simulink model "systemTest"  (R2014a)
settings: Solver=ode45  StartTime=0.0  StopTime=100  RelTol=1e-3
values from neighbouring files (symbols this model uses):
  friX1 = 4    [parameters1.m]
  friX2 = 0.76462    [parameters1.m]
  friY = 8    [parameters1.m]
  friZ = 4    [parameters1.m]
  I = 1/12*m*((2*ry1)^2 + (2*rx1)^2)    (= 7.53502955357)    [parameters1.m]
  inputBound = [minInput maxInput]    [parameters1.m]
  K = [1000 1000 1000 10 10 1 1]    [parameters1.m]
  k1m = 50    [parameters1.m]
  k1x = 100    [parameters1.m]
  k1y = 100    [parameters1.m]
  k2m = 25    [parameters1.m]
  k2x = 60    [parameters1.m]
  k2y = 60    [parameters1.m]
  m = 46.27    [parameters1.m]
  rx1 = rx01    [Minimizer.m]    (also in parameters1.m = -0.635)
  rx2 = rx02    [Minimizer.m]    (also in parameters1.m = -0.635)
  ry1 = ry01    [Minimizer.m]    (also in parameters1.m = 0.2921)
  ry2 = ry02    [Minimizer.m]    (also in parameters1.m = -0.2921)
settings Model: Creator=propagator  LastModifiedBy=propagator

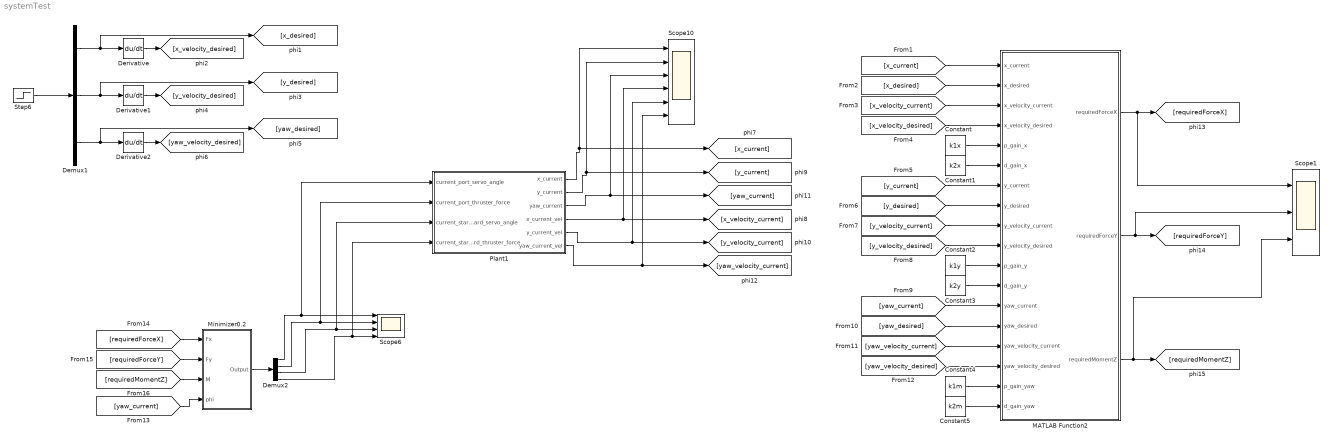
== system systemTest ==
  Constant : Constant  Value=k1x
  Constant1 : Constant  Value=k2x
  Constant2 : Constant  Value=k1y
  Constant3 : Constant  Value=k2y
  Constant4 : Constant  Value=k1m
  Constant5 : Constant  Value=k2m
  Demux1 : Demux  Outputs=3
  Demux2 : Demux
  Derivative : Derivative
  Derivative1 : Derivative
  Derivative2 : Derivative
  MATLAB Function2 : MATLAB Function  TreatAsAtomicUnit=on
  Minimizer0.2 : Subsystem  mask{rx1=rx1, rx2=rx2, ry1=ry1, ry2=ry2, C=K, inputBound=inputBound, m=m, I=I}
      mask prompts: C "Performance Gain"; inputBound "Input Bounds"; m "Boat Mass"; I "Boat Inertia"
      mask TypeOptions m: Constant6/Value
      mask TypeOptions I: Constant7/Value
  Plant1 : Subsystem  mask{rx1=rx1, ry1=ry1, ry2=ry2, M=m, I=I, friX1=friX1, friX2=friX2, friY=friY, friZ=friZ}
      mask TypeOptions rx1: Constant/Value
      mask TypeOptions friX1: Constant1/Value
      mask TypeOptions friX2: Constant8/Value
      mask TypeOptions friY: Constant7/Value
      mask TypeOptions friZ: Constant9/Value
  Scope1 : Scope  NumInputPorts=3
      settings: YMin=-3~905~-185  YMax=0~940~-155
  Scope10 : Scope  NumInputPorts=6
      settings: YMin=1.83~5.87~12~0.03265~0.0811~-0.1116  YMax=1.87~5.97~12.13~0.03305~0.08155~-0.1103  SaveName=ScopeData9
  Scope6 : Scope  NumInputPorts=4
      settings: YMin=-1~-23~45.5556~25  YMax=1~-23~45.5556~32.5  SaveName=ScopeData5
  Step6 : Step  Before=[0;0;0]  After=[0;10;0]  SampleTime=0
  wires:
  Demux2/1 -> Plant1/1(current_port_servo_angle), Scope6/1
  Demux2/2 -> Plant1/2(current_port_thruster_force), Scope6/2
  Demux2/3 -> Plant1/3(current_starboard_servo_angle), Scope6/3
  Demux2/4 -> Plant1/4(current_starboard_thruster_force), Scope6/4
  Minimizer0.2/1(Output) -> Demux2/1
  Constant1/1 -> MATLAB Function2/6(d_gain_x)
  Constant/1 -> MATLAB Function2/5(p_gain_x)
  Constant4/1 -> MATLAB Function2/17(p_gain_yaw)
  Constant5/1 -> MATLAB Function2/18(d_gain_yaw)
  Constant3/1 -> MATLAB Function2/12(d_gain_y)
  Constant2/1 -> MATLAB Function2/11(p_gain_y)
  [x_current] -> MATLAB Function2/1(x_current)
  [x_desired] -> MATLAB Function2/2(x_desired)
  [x_velocity_current] -> MATLAB Function2/3(x_velocity_current)
  [x_velocity_desired] -> MATLAB Function2/4(x_velocity_desired)
  [yaw_velocity_desired] -> MATLAB Function2/16(yaw_velocity_desired)
  [yaw_velocity_current] -> MATLAB Function2/15(yaw_velocity_current)
  [yaw_desired] -> MATLAB Function2/14(yaw_desired)
  [yaw_current] -> MATLAB Function2/13(yaw_current)
  [y_velocity_desired] -> MATLAB Function2/10(y_velocity_desired)
  [y_velocity_current] -> MATLAB Function2/9(y_velocity_current)
  [y_desired] -> MATLAB Function2/8(y_desired)
  [y_current] -> MATLAB Function2/7(y_current)
  Demux1/3 -> [yaw_desired], Derivative2/1
  Demux1/2 -> [y_desired], Derivative1/1
  Derivative2/1 -> [yaw_velocity_desired]
  Derivative1/1 -> [y_velocity_desired]
  Demux1/1 -> [x_desired], Derivative/1
  Step6/1 -> Demux1/1
  Derivative/1 -> [x_velocity_desired]
  Plant1/1(x_current) -> Scope10/1, [x_current]
  Plant1/2(y_current) -> Scope10/2, [y_current]
  Plant1/6(yaw_current_vel) -> Scope10/6, [yaw_velocity_current]
  Plant1/3(yaw_current) -> Scope10/3, [yaw_current]
  Plant1/4(x_current_vel) -> Scope10/4, [x_velocity_current]
  Plant1/5(y_current_vel) -> Scope10/5, [y_velocity_current]
  MATLAB Function2/2(requiredForceY) -> Scope1/2, [requiredForceY]
  MATLAB Function2/3(requiredMomentZ) -> Scope1/3, [requiredMomentZ]
  MATLAB Function2/1(requiredForceX) -> Scope1/1, [requiredForceX]
  [yaw_current] -> Minimizer0.2/4(phi)
  [requiredMomentZ] -> Minimizer0.2/3(M)
  [requiredForceY] -> Minimizer0.2/2(Fy)
  [requiredForceX] -> Minimizer0.2/1(Fx)

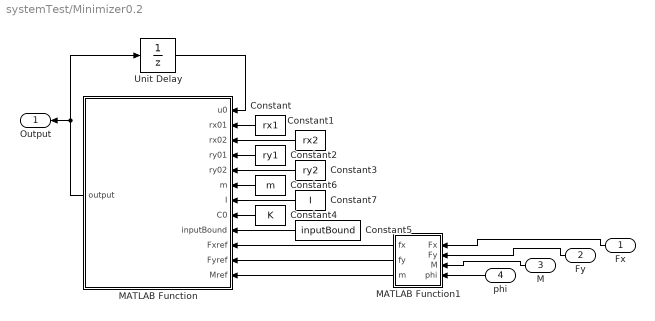
== system systemTest/Minimizer0.2 ==
  Fx : Inport
  Fy : Inport  Port=2
  M : Inport  Port=3
  phi : Inport  Port=4
  Constant : Constant  Value=rx1
  Constant1 : Constant  Value=rx2
  Constant2 : Constant  Value=ry1
  Constant3 : Constant  Value=ry2
  Constant4 : Constant  Value=K
  Constant5 : Constant  Value=inputBound
  Constant6 : Constant  Value=m
  Constant7 : Constant  Value=I
  MATLAB Function : MATLAB Function  TreatAsAtomicUnit=on
  MATLAB Function1 : MATLAB Function  TreatAsAtomicUnit=on
  Unit Delay : UnitDelay  InitialCondition=[0;0;0;0]  SampleTime=-1
  Output : Outport
  wires:
  Constant/1 -> MATLAB Function/2(rx01)
  Constant1/1 -> MATLAB Function/3(rx02)
  Constant2/1 -> MATLAB Function/4(ry01)
  Constant4/1 -> MATLAB Function/8(C0)
  Unit Delay/1 -> MATLAB Function/1(u0)
  MATLAB Function/1(output) -> Unit Delay/1, Output/1
  Constant5/1 -> MATLAB Function/9(inputBound)
  Constant3/1 -> MATLAB Function/5(ry02)
  MATLAB Function1/3(m) -> MATLAB Function/12(Mref)
  MATLAB Function1/2(fy) -> MATLAB Function/11(Fyref)
  MATLAB Function1/1(fx) -> MATLAB Function/10(Fxref)
  Fy/1 -> MATLAB Function1/2(Fy)
  Fx/1 -> MATLAB Function1/1(Fx)
  M/1 -> MATLAB Function1/3(M)
  phi/1 -> MATLAB Function1/4(phi)
  Constant6/1 -> MATLAB Function/6(m)
  Constant7/1 -> MATLAB Function/7(I)

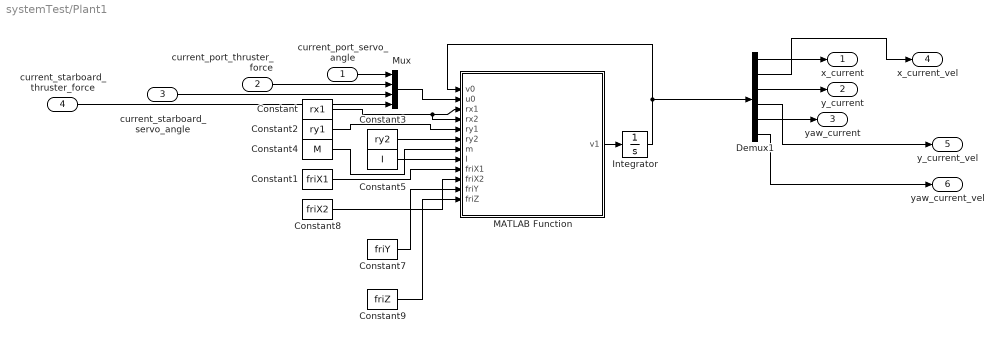
== system systemTest/Plant1 ==
  current_port_servo_angle : Inport
  current_port_thruster_force : Inport  Port=2
  current_starboard_servo_angle : Inport  Port=3
  current_starboard_thruster_force : Inport  Port=4
  Constant : Constant  Value=rx1
  Constant1 : Constant  Value=friX1
  Constant2 : Constant  Value=ry1
  Constant3 : Constant  Value=ry2
  Constant4 : Constant  Value=M
  Constant5 : Constant  Value=I
  Constant7 : Constant  Value=friY
  Constant8 : Constant  Value=friX2
  Constant9 : Constant  Value=friZ
  Demux1 : Demux  Outputs=6
  Integrator : Integrator  InitialCondition=[0 0 0 0 0 0]
  MATLAB Function : MATLAB Function  TreatAsAtomicUnit=on
  Mux : Mux
  x_current : Outport
  y_current : Outport  Port=2
  yaw_current : Outport  Port=3
  x_current_vel : Outport  Port=4
  y_current_vel : Outport  Port=5
  yaw_current_vel : Outport  Port=6
  wires:
  Constant/1 -> MATLAB Function/3(rx1), MATLAB Function/4(rx2)
  Constant2/1 -> MATLAB Function/5(ry1)
  Constant3/1 -> MATLAB Function/6(ry2)
  Constant4/1 -> MATLAB Function/7(m)
  Constant5/1 -> MATLAB Function/8(I)
  MATLAB Function/1(v1) -> Integrator/1
  Integrator/1 -> MATLAB Function/1(v0), Demux1/1
  current_port_servo_angle/1 -> Mux/1
  current_port_thruster_force/1 -> Mux/2
  current_starboard_servo_angle/1 -> Mux/3
  current_starboard_thruster_force/1 -> Mux/4
  Mux/1 -> MATLAB Function/2(u0)
  Constant1/1 -> MATLAB Function/9(friX1)
  Constant7/1 -> MATLAB Function/11(friY)
  Constant9/1 -> MATLAB Function/12(friZ)
  Constant8/1 -> MATLAB Function/10(friX2)
  Demux1/5 -> yaw_current/1
  Demux1/3 -> y_current/1
  Demux1/1 -> x_current/1
  Demux1/2 -> x_current_vel/1
  Demux1/4 -> y_current_vel/1
  Demux1/6 -> yaw_current_vel/1

== matlab function systemTest/MATLAB Function2 ==
  data: x_current input; requiredForceX output; x_desired input; x_velocity_current input; x_velocity_desired input; p_gain_x input; d_gain_x input; y_current input; y_desired input; y_velocity_current input; y_velocity_desired input; p_gain_y input; d_gain_y input; yaw_current input; yaw_desired input; yaw_velocity_current input; yaw_velocity_desired input; p_gain_yaw input; d_gain_yaw input; requiredForceY output; requiredMomentZ output
function [requiredForceX,requiredForceY,requiredMomentZ] = fcn(x_current,x_desired,x_velocity_current,x_velocity_desired, p_gain_x,d_gain_x,...
                            y_current,y_desired,y_velocity_current,y_velocity_desired, p_gain_y, d_gain_y,...
                            yaw_current,yaw_desired,yaw_velocity_current,yaw_velocity_desired, p_gain_yaw, d_gain_yaw)

requiredForceX = p_gain_x * (x_desired - x_current) + d_gain_x * (x_velocity_desired - x_velocity_current);
requiredForceY = p_gain_y * (y_desired - y_current) + d_gain_y * (y_velocity_desired - y_velocity_current);
requiredMomentZ = p_gain_yaw * (yaw_desired - yaw_current) + d_gain_yaw * (yaw_velocity_desired - yaw_velocity_current);
end

== matlab function systemTest/Plant1/MATLAB Function ==
  data: v0 input; v1 output; u0 input; rx1 input; rx2 input; ry1 input; ry2 input; m input; I input; friX1 input; friX2 input; friY input; friZ input

function v1   = boatDynamics(v0, u0, rx1, rx2, ry1, ry2, m, I, friX1,friX2, friY, friZ)

    % %%%%%%%%%%%%%%%%%%%%%%%%%%%%%%%%%%%%%%%%%%%% %
    %    v = [x...          %    u = [theta1...    %
    %        x_dot...       %        f1...         %
    %        y...           %        theta2...     %
    %        y_dot...       %        f2]           %
    %        theta...       %                      %
    %        theta_dot];    %                      %
    % %%%%%%%%%%%%%%%%%%%%%%%%%%%%%%%%%%%%%%%%%%%% %
    
    v11 = v0(2);
    v12 = u0(2)/m*cosd(u0(1)+v0(5)) + u0(4)/m*cosd(u0(3)+v0(5)) - (friX1*v0(2)*(cosd(v0(5))+sind(v0(5))) - friX2*(v0(2)*(cosd(v0(5))+sind(v0(5))))^2);
    v13 = v0(4);
    v14 = u0(2)/m*sind(u0(1)+v0(5)) + u0(4)/m*sind(u0(3)+v0(5)) - friY*v0(4)*(-sind(v0(5))+cosd(v0(5)));
    v15 = v0(6);
    v16 = -rx1/I*u0(2)*sind(u0(1)) + ry1/I*u0(2)*cosd(u0(1)) - rx2/I*u0(4)*sind(u0(3)) + ry2/I*u0(4)*cosd(u0(3)) - friZ*v0(6);
   
    v1 = [v11;v12;v13;v14;v15;v16];
    
end

== matlab function systemTest/Minimizer0.2/MATLAB Function ==
  data: u0 input; output output; rx01 input; rx02 input; ry01 input; ry02 input; m input; I input; C0 input; inputBound input; Fxref input; Fyref input; Mref input
function output = Minimizer(u0, rx01, rx02, ry01, ry02, m, I, C0, inputBound, Fxref, Fyref, Mref)

rx1 = rx01; rx2 = rx02;
ry1 = ry01; ry2 = ry02;

C = C0;

%Fxref = Fx; Fyref = Fy; Mref  = M;

gridNum = 10;

grid = boundGrid(inputBound, gridNum, rx1,ry1);

u1 = getMinFromGrid(grid, u0, Fxref, Fyref, Mref, rx1, rx2, ry1, ry2, C, m, I);

% u1 = u0;

% %     for k = 1:20
% %         h = getDirection(u1, u0, Fxref, Fyref, Mref, rx1, rx2, ry1, ry2, C);
% %         alpha = getStepSize(u1, u0, h, Fxref, Fyref, Mref, rx1, rx2, ry1, ry2, C);
% %         u1 = u1 + alpha*h;
% %         u1 = checkInputBound(u1,inputBound);
% %     end
    
    output = u1;

end

function output = getMinFromGrid(grid, preinput, Fxref, Fyref, Mref, rx1, rx2, ry1, ry2, C, m, I)

[ii, iii] = size(grid);
v0 = costFunction(grid(1,:), preinput, Fxref, Fyref, Mref, rx1, rx2, ry1, ry2, C, m, I);

output = [grid(1,1);grid(1,2);grid(1,3);grid(1,4)];

for i = 1:ii
    for j = 1:ii
        for k = 1:ii
            for l = 1:ii
                input = [grid(i,1);grid(j,2);grid(k,3);grid(l,4)];
                v1 = costFunction(input,preinput, Fxref, Fyref, Mref, rx1, rx2, ry1, ry2, C, m, I);
                if v0 > v1
                    v0 = v1;
                    output = input;
                else
                end
            end
        end
    end
end

end

function output = checkInputBound(input,inputBound)
k = [0;0;0;0];
    for i = 1:length(input)
        k(i) = sat(input(i),inputBound(i,:));
    end
    output = k;
end

function output = boundGrid(inputBound, gridNum, rx1,ry1)

p = gridNum;

theta1 =    linspace(inputBound(1,1),inputBound(1,2),p)';
f1 =        linspace(inputBound(2,1),inputBound(2,2),p)';
theta2 =    linspace(inputBound(3,1),inputBound(3,2),p)';
f2 =        linspace(inputBound(4,1),inputBound(4,2),p)';

%i = atan(rx1/ry1)*180/pi;

output = [theta1, f1, theta2, f2;...
          0,  0,      0,  0];
%             i,    0,    i,    0];

end

function output = sat(input, bound)

    if input < bound(1)
        output = bound(1);
    elseif input > bound(2)
        output = bound(2);
    else
        output = input;
    end

end

function output = getStepSize(input, preinput, h, Fxref, Fyref, Mref, rx1, rx2, ry1, ry2, C, m, I)

    alpha = .001;
    
    u0 = input;
    u1 = input + alpha*h;
    
    v0 = costFunction( u0, preinput, Fxref, Fyref, Mref, rx1, rx2, ry1, ry2, C, m, I );
    v1 = costFunction( u1, preinput, Fxref, Fyref, Mref, rx1, rx2, ry1, ry2, C, m, I);

    while v1 <= v0 && v1 ~= 0
        alpha = alpha + .001;
        u1 = input + alpha*h;
        v0 = v1;
        v1 = costFunction( u1, preinput, Fxref, Fyref, Mref, rx1, rx2, ry1, ry2, C, m, I );
    end
    
    v0 = v1;
    alpha = .0015;

    while v1 <= v0  && v1 ~= 0
        alpha = alpha - 0.0001;
        u1 = input + alpha*h;
        v0 = v1;
        v1 = costFunction( u1, preinput, Fxref, Fyref, Mref, rx1, rx2, ry1, ry2, C, m, I );
    end


    output = alpha;

end

function output = costFunction(input, preinput, Fxref, Fyref, Mref, rx1, rx2, ry1, ry2, C, m, I)

    theta1  = input(1);
    f1      = input(2);
    theta2  = input(3);
    f2      = input(4);
    
    pretheta1   = preinput(1);
    pretheta2   = preinput(3);

    Fx = f1*cosd(theta1) + f2*cosd(theta2);
    Fy = f1*sind(theta1) + f2*sind(theta2);
    M = -rx1*f1*sind(theta1) + ry1*f1*cosd(theta1) - rx2*f2*sind(theta2)...
        + ry2*f2*cosd(theta2);

    output = C(1)*(Fx-Fxref)^2 +...
        C(2)*(Fy-Fyref)^2 +...
        C(3)*(M-Mref)^2  +...
        C(4)*f1^2 +...
        C(5)*f2^2 +...
        C(6)*(theta1 - pretheta1)^2 +...
        C(7)*(theta2 - pretheta2)^2;% +...
%         C(5)*theta1^2 +...
%         C(5)*theta2^2;

end

function output = getDirection(input, preinput, Fxref, Fyref, Mref, rx1, rx2, ry1, ry2, C, m, I)

hsd = SteepestDescent(input, preinput, Fxref, Fyref, Mref, rx1, rx2, ry1, ry2, C, m, I);

output = zeros(4,1);

    for i = 1:length(hsd)
        output(i) = hsd(i);
    end
    
end

function output = SteepestDescent(input, preinput, Fxref, Fyref, Mref, rx1, rx2, ry1, ry2, C, m, I)

theta1  = input(1);
f1      = input(2);
theta2  = input(3);
f2      = input(4);

pretheta1   = preinput(1);
pretheta2   = preinput(3);

dVdtheta1 = C(3)*(f1*ry1*cosd(theta1)...
    - f1*rx1*sind(theta1))*(f1*rx1*cosd(theta1)...
    - Mref + f2*rx2*cosd(theta2) + f1*ry1*sin(theta1)...
    + f2*ry2*sind(theta2)) - C(6)*(pretheta1 - theta1)...
    - C(2)*f1*sind(theta1)*(f1*cosd(theta1) - Fyref + f2*cosd(theta2))...
    + C(1)*f1*cosd(theta1)*(Fxref + f1*sind(theta1) + f2*sind(theta2));

dVdf1 = C(4)*f1 + C(1)*sind(theta1)*(Fxref + f1*sin(theta1)...
    + f2*sind(theta2)) + C(2)*cosd(theta1)*(f1*cosd(theta1) - Fyref...
    + f2*cosd(theta2)) + C(3)*(rx1*cosd(theta1)...
    + ry1*sind(theta1))*(f1*rx1*cosd(theta1) - Mref + f2*rx2*cosd(theta2)...
    + f1*ry1*sind(theta1) + f2*ry2*sind(theta2));

dVdtheta2 = C(3)*(f2*ry2*cosd(theta2)...
    - f2*rx2*sind(theta2))*(f1*rx1*cosd(theta1)...
    - Mref + f2*rx2*cosd(theta2) + f1*ry1*sind(theta1)...
    + f2*ry2*sind(theta2)) - C(7)*(pretheta2 - theta2)...
    - C(2)*f2*sind(theta2)*(f1*cosd(theta1) - Fyref + f2*cosd(theta2))...
    + C(1)*f2*cosd(theta2)*(Fxref + f1*sind(theta1) + f2*sind(theta2));

dVdf2 = C(5)*f2 + C(1)*sind(theta2)*(Fxref + f1*sind(theta1)...
    + f2*sind(theta2)) + C(2)*cosd(theta2)*(f1*cosd(theta1) - Fyref...
    + f2*cosd(theta2)) + C(3)*(rx2*cosd(theta2)...
    + ry2*sind(theta2))*(f1*rx1*cosd(theta1) - Mref + f2*rx2*cosd(theta2)...
    + f1*ry1*sind(theta1) + f2*ry2*sind(theta2));
 
output = -[dVdtheta1; dVdf1; dVdtheta2; dVdf2];

end

== matlab function systemTest/Minimizer0.2/MATLAB Function1 ==
  data: Fx input; fx output; Fy input; M input; fy output; m output; phi input
function [fx,fy,m] = fcn(Fx,Fy,M, phi)
%#codegen

R = [cosd(phi) -sind(phi) 0;...
        sind(phi)  cosd(phi) 0;...
        0           0       1];
    
    FxyM = R'*[Fx;Fy;M];
    
    fx = FxyM(1);
    fy = FxyM(2);
    m = FxyM(3);
    
end
